simulink model "test_flock_gazebo"  (R2023b)
settings: Solver=FixedStepAuto  StartTime=0.0  StopTime=inf  RelTol=1e-3
values from neighbouring files (symbols this model uses):
  a = 1    [main_flock3.m]    (also in main_flock4.m; params_flocking_ros.m)
  b = 1    [main_flock3.m]    (also in main_flock4.m; params_flocking_ros.m)
  c = 1    [main_flock3.m]    (also in main_flock4.m; params_flocking_ros.m)
  c_gammap = 1.2    [main_flock3.m]    (also in main_flock4.m)
  c_gammav = 3.5    [main_flock3.m]    (also in main_flock4.m)
  d = 0.6    [main_flock3.m]    (also in main_flock4.m; params_flocking_ros.m)
  d_prime = 1    [main_flock3.m]    (also in main_flock4.m; params_flocking_ros.m)
  epsilon = 0.1    [main_flock3.m]    (also in main_flock4.m; params_flocking_ros.m)
  h = 0.2    [main_flock3.m]    (also in main_flock4.m; params_flocking_ros.m)
  R = 0.15    [main_flock3.m]    (also in main_flock4.m; params_flocking_ros.m)
  vxobs = 0    [main_flock3.m]    (also in main_flock4.m)
  vyobs = 0    [main_flock3.m]    (also in main_flock4.m)
  vzobs = 0    [main_flock3.m]    (also in main_flock4.m)
  xmax = 2    [main_flock3.m]    (also in main_flock4.m)
  xmin = -2    [main_flock3.m]    (also in main_flock4.m)
  xobs = 0.75    [main_flock3.m]    (also in main_flock4.m)
  yobs = -0.25    [main_flock3.m]    (also in main_flock4.m)
  zobs = 1.7    [main_flock3.m]    (also in main_flock4.m)
undefined symbols (not defined in the file or in its folder): angular, DiscIntNeverNeededParam, linear
libraries: ros2lib x14, robotcorelib x4
(part 1 of 2)
settings Model: Creator=johvany  LastModifiedBy=jonatan_alvarez
settings OptimizationCC: EnhancedBackFolding=on  PassReuseOutputArgsThreshold=0  ZeroExternalMemoryAtStartup=off  ZeroInternalMemoryAtStartup=off  MaxStackSize=64  OptimizeBlockOrder=speed  DifferentSizesBufferReuse=on  OptimizationCustomize=off
settings DebuggingCC: ParameterTunabilityLossMsg=error
settings HardwareCC: ProdBitPerLong=64  ProdHWDeviceType=Intel->x86-64 (Linux 64)  UseEmbeddedCoderFeatures=off
settings SFSimCC: MATLABDynamicMemAlloc=off
settings RTWCC: Description=Embedded Coder  SystemTargetFile=ert.tlc  HardwareBoard=Robot Operating System 2 (ROS 2)  TLCOptions="-aInlineSetEventsForThisBaseRateFcn=TLC_FALSE -aSuppressMultiTaskScheduler=TLC_FALSE  -aRateBasedStepFcn=0"  TemplateMakefile=ert_default_tmf  Toolchain=Colcon Tools  TargetLang=C++
settings CodeAppCC: ForceParamTrailComments=on  OperatorAnnotations=on
settings ERTTargetCC: ERTCustomFileBanners=off  CodeInterfacePackaging=C++ class  SupportContinuousTime=on  SupportNonInlinedSFcns=on  RemoveResetFunc=off  ModelStepFunctionPrototypeControlCompliant=off  RootIOFormat=Structure reference

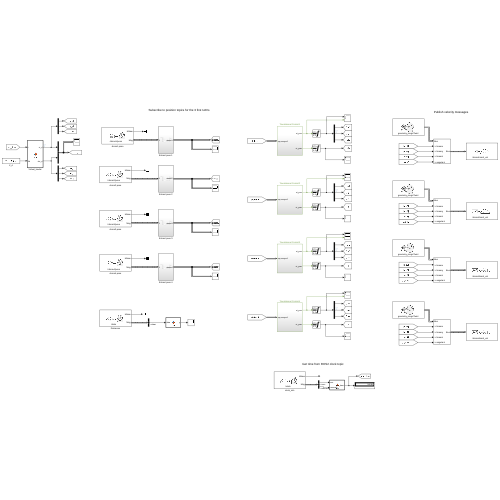
[thumbnail: Simulink's stored preview of the top-level diagram]
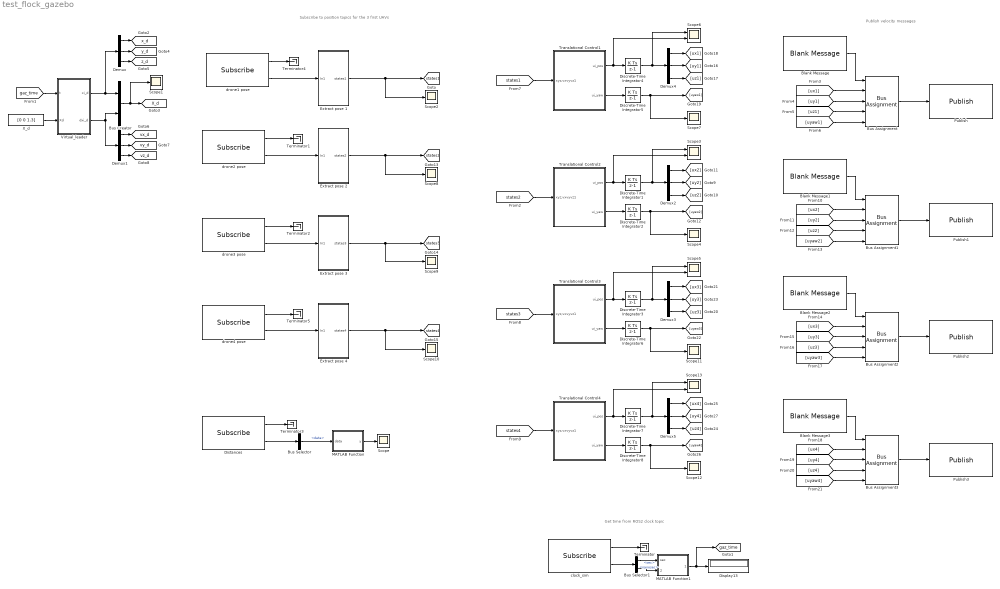
== system test_flock_gazebo ==
  note: Publish velocity messages
  note: Subscribe to position topics for the 3 first UAVs
  note: Get time from ROS2 clock topic
  Blank Message{,1..3} (4 alike) : ros2lib/Blank Message  messageClass=Message  entityType=geometry_msgs/Twist  messageType=geometry_msgs/Twist  SampleTime=inf
  Bus Assignment{,1..3} (4 alike) : BusAssignment  AssignedSignals=linear.x,linear.y,linear.z,angular.z
  Bus Creator : BusCreator  Inputs=2
  Bus Selector : BusSelector  OutputSignals=data
  Bus Selector1 : BusSelector  OutputSignals=clock.sec,clock.nanosec
  Demux{,1..5} (6 alike) : Demux  Outputs=3
  Discrete-Time Integrator{1..8} (8 alike) : DiscreteIntegrator  SampleTime=-1  LimitOutput=on  UpperSaturationLimit=5  LowerSaturationLimit=-5  ICPrevOutput=DiscIntNeverNeededParam  ICPrevScaledInput=DiscIntNeverNeededParam
  Display13 : Display
      settings: Decimation=4
  Distances : ros2lib/Subscribe  topicSource=Select from ROS network  topic=/dists  messageType=std_msgs/Float32MultiArray  sampleTime=-1  QOSHistory=Keep last  QOSDepth=1  QOSReliability=Reliable  QOSDurability=Volatile
  Extract pose 1 : Subsystem
  Extract pose 2 : Subsystem
  Extract pose 3 : Subsystem
  Extract pose 4 : Subsystem
  MATLAB Function : MATLAB Function  TreatAsAtomicUnit=on
  MATLAB Function1 : MATLAB Function  TreatAsAtomicUnit=on
  Publish : ros2lib/Publish  topicSource=Select from ROS network  topic=/drone1/cmd_vel  messageType=geometry_msgs/Twist  QOSHistory=Keep last  QOSDepth=1  QOSReliability=Reliable  QOSDurability=Volatile
  Publish1 : ros2lib/Publish  topicSource=Select from ROS network  topic=/drone2/cmd_vel  messageType=geometry_msgs/Twist  QOSHistory=Keep last  QOSDepth=1  QOSReliability=Reliable  QOSDurability=Volatile
  Publish2 : ros2lib/Publish  topicSource=Select from ROS network  topic=/drone3/cmd_vel  messageType=geometry_msgs/Twist  QOSHistory=Keep last  QOSDepth=1  QOSReliability=Reliable  QOSDurability=Volatile
  Publish3 : ros2lib/Publish  topicSource=Select from ROS network  topic=/drone4/cmd_vel  messageType=geometry_msgs/Twist  QOSHistory=Keep last  QOSDepth=1  QOSReliability=Reliable  QOSDurability=Volatile
  Scope{,1..2,4,7..12} (10 alike) : Scope
  Scope{3,5..6,13} (4 alike) : Scope  NumInputPorts=2
  Terminator{,1..5} (6 alike) : Terminator
  Translational Control1 : Subsystem
  Translational Control2 : Subsystem
  Translational Control3 : Subsystem
  Translational Control4 : Subsystem
  Virtual_leader : MATLAB Function  TreatAsAtomicUnit=on
  X_d : Constant  Value=[0 0 1.3]
  clock_sim : ros2lib/Subscribe  topicSource=Select from ROS network  topic=/clock  messageType=rosgraph_msgs/Clock  sampleTime=-1  QOSHistory=Keep last  QOSDepth=1  QOSReliability=Reliable  QOSDurability=Volatile
  drone1 pose : ros2lib/Subscribe  topicSource=Select from ROS network  topic=/drone1/pose  messageType=geometry_msgs/PoseStamped  sampleTime=-1  QOSHistory=Keep last  QOSDepth=1  QOSReliability=Reliable  QOSDurability=Volatile
  drone2 pose : ros2lib/Subscribe  topicSource=Select from ROS network  topic=/drone2/pose  messageType=geometry_msgs/PoseStamped  sampleTime=-1  QOSHistory=Keep last  QOSDepth=1  QOSReliability=Reliable  QOSDurability=Volatile
  drone3 pose : ros2lib/Subscribe  topicSource=Select from ROS network  topic=/drone3/pose  messageType=geometry_msgs/PoseStamped  sampleTime=-1  QOSHistory=Keep last  QOSDepth=1  QOSReliability=Reliable  QOSDurability=Volatile
  drone4 pose : ros2lib/Subscribe  topicSource=Select from ROS network  topic=/drone4/pose  messageType=geometry_msgs/PoseStamped  sampleTime=-1  QOSHistory=Keep last  QOSDepth=1  QOSReliability=Reliable  QOSDurability=Volatile
  tag scope: X_d=global, gaz_time=global, states1=global, states2=global, states3=global, states4=global, vx_d=global, vy_d=global, vz_d=global, x_d=global, y_d=global, z_d=global
  wires:
  clock_sim/1 -> Terminator/1
  drone2 pose/2 -> Extract pose 2/1(In1)
  drone2 pose/1 -> Terminator1/1
  drone3 pose/2 -> Extract pose 3/1(In1)
  drone3 pose/1 -> Terminator2/1
  Blank Message/1 -> Bus Assignment/1
  Bus Assignment/1 -> Publish/1
  Blank Message1/1 -> Bus Assignment1/1
  Bus Assignment1/1 -> Publish1/1
  Blank Message2/1 -> Bus Assignment2/1
  Bus Assignment2/1 -> Publish2/1
  Blank Message3/1 -> Bus Assignment3/1
  Bus Assignment3/1 -> Publish3/1
  Distances/1 -> Terminator3/1
  Distances/2 -> Bus Selector/1
  Bus Selector/1 -> MATLAB Function/1(data)  "<data>"
  MATLAB Function/1(y) -> Scope/1
  clock_sim/2 -> Bus Selector1/1
  Bus Selector1/1 -> MATLAB Function1/1(sec)  "<sec>"
  Bus Selector1/2 -> MATLAB Function1/2(nanosec)  "<nanosec>"
  Demux1/1 -> [vx_d]
  Demux1/3 -> [vz_d]
  Demux/1 -> [x_d]
  Demux/2 -> [y_d]
  Virtual_leader/2(dxi_d) -> Bus Creator/2, Demux1/1
  Bus Creator/1 -> Scope1/1, [X_d]
  Demux1/2 -> [vy_d]
  [gaz_time] -> Virtual_leader/1(t)
  Demux/3 -> [z_d]
  Virtual_leader/1(xi_d) -> Demux/1, Bus Creator/1
  drone1 pose/1 -> Terminator4/1
  drone1 pose/2 -> Extract pose 1/1(In1)
  MATLAB Function1/1(gaz_time) -> [gaz_time], Display13/1
  Extract pose 1/1(states1) -> [states1], Scope2/1
  [ux1] -> Bus Assignment/2
  [uy1] -> Bus Assignment/3
  [uz1] -> Bus Assignment/4
  [uyaw1] -> Bus Assignment/5
  X_d/1 -> Virtual_leader/2(Xd)
  [states1] -> Translational Control1/1(xyz,vxvyvz1)
  Translational Control1/1(ui_pos) -> Scope6/2, Discrete-Time Integrator4/1
  Translational Control1/2(ui_yaw) -> Discrete-Time Integrator5/1
  Discrete-Time Integrator5/1 -> [uyaw1], Scope7/1
  Extract pose 2/1(states2) -> Scope8/1, [states2]
  Extract pose 3/1(states3) -> [states3], Scope9/1
  Extract pose 4/1(states4) -> Scope10/1, [states4]
  drone4 pose/1 -> Terminator5/1
  drone4 pose/2 -> Extract pose 4/1(In1)
  Demux4/1 -> [ux1]
  Demux4/3 -> [uz1]
  Demux4/2 -> [uy1]
  Discrete-Time Integrator4/1 -> Scope6/1, Demux4/1
  Discrete-Time Integrator1/1 -> Demux2/1, Scope3/1
  Demux2/2 -> [uy2]
  Demux2/3 -> [uz2]
  Demux2/1 -> [ux2]
  Discrete-Time Integrator2/1 -> Scope4/1, [uyaw2]
  Translational Control2/2(ui_yaw) -> Discrete-Time Integrator2/1
  Translational Control2/1(ui_pos) -> Discrete-Time Integrator1/1, Scope3/2
  [states2] -> Translational Control2/1(xyz,vxvyvz1)
  [states3] -> Translational Control3/1(xyz,vxvyvz1)
  Translational Control3/1(ui_pos) -> Scope5/2, Discrete-Time Integrator3/1
  Translational Control3/2(ui_yaw) -> Discrete-Time Integrator6/1
  Discrete-Time Integrator6/1 -> [uyaw3], Scope11/1
  Demux3/1 -> [ux3]
  Demux3/3 -> [uz3]
  Demux3/2 -> [uy3]
  Discrete-Time Integrator3/1 -> Scope5/1, Demux3/1
  Discrete-Time Integrator7/1 -> Demux5/1, Scope13/1
  Demux5/2 -> [uy4]
  Demux5/3 -> [uz4]
  Demux5/1 -> [ux4]
  Discrete-Time Integrator8/1 -> Scope12/1, [uyaw4]
  Translational Control4/2(ui_yaw) -> Discrete-Time Integrator8/1
  Translational Control4/1(ui_pos) -> Discrete-Time Integrator7/1, Scope13/2
  [states4] -> Translational Control4/1(xyz,vxvyvz1)
  [ux2] -> Bus Assignment1/2
  [uy2] -> Bus Assignment1/3
  [uz2] -> Bus Assignment1/4
  [uyaw2] -> Bus Assignment1/5
  [uyaw3] -> Bus Assignment2/5
  [uz3] -> Bus Assignment2/4
  [uy3] -> Bus Assignment2/3
  [ux3] -> Bus Assignment2/2
  [ux4] -> Bus Assignment3/2
  [uy4] -> Bus Assignment3/3
  [uz4] -> Bus Assignment3/4
  [uyaw4] -> Bus Assignment3/5

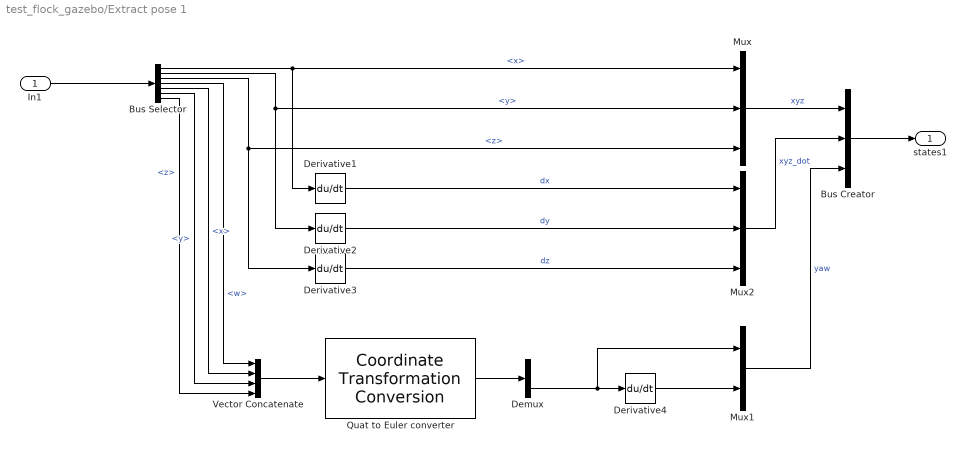
== system test_flock_gazebo/Extract pose 1 ==
  In1 : Inport
  Bus Creator : BusCreator  Inputs=3
  Bus Selector : BusSelector  OutputSignals=pose.position.x,pose.position.y,pose.position.z,pose.orientation.w,pose.orientation.x,pose.orientation.y,pose.orientation.z
  Demux : Demux  Outputs=3
  Derivative{1..4} (4 alike) : Derivative
  Mux : Mux  Inputs=3
  Mux1 : Mux  Inputs=2
  Mux2 : Mux  Inputs=3
  Quat to Euler converter : robotcorelib/Coordinate Transformation Conversion  InputRepresentation=Quaternion  InputEulerSequence=ZYX  ShowTrVecInputPort=on  OutputRepresentation=Euler Angles  OutputEulerSequence=XYZ  ShowTrVecOutputPort=on  SimulateUsing=Interpreted execution
      settings: LibrarySourceBlock=roslib/Utilities/Coordinate Transformation Conversion
  Vector Concatenate : Concatenate  NumInputs=4
  states1 : Outport
  wires:
  Bus Selector/5 -> Vector Concatenate/2  "<x>"
  Quat to Euler converter/1 -> Demux/1
  Demux/3 -> Mux1/1, Derivative4/1
  Bus Selector/6 -> Vector Concatenate/3  "<y>"
  Bus Selector/1 -> Derivative1/1, Mux/1  "<x>"
  Bus Selector/7 -> Vector Concatenate/4  "<z>"
  Vector Concatenate/1 -> Quat to Euler converter/1
  In1/1 -> Bus Selector/1
  Bus Selector/4 -> Vector Concatenate/1  "<w>"
  Bus Selector/2 -> Derivative2/1, Mux/2  "<y>"
  Bus Selector/3 -> Derivative3/1, Mux/3  "<z>"
  Derivative4/1 -> Mux1/2
  Bus Creator/1 -> states1/1
  Derivative1/1 -> Mux2/1  "dx"
  Derivative2/1 -> Mux2/2  "dy"
  Derivative3/1 -> Mux2/3  "dz"
  Mux/1 -> Bus Creator/1  "xyz"
  Mux2/1 -> Bus Creator/2  "xyz_dot"
  Mux1/1 -> Bus Creator/3  "yaw"

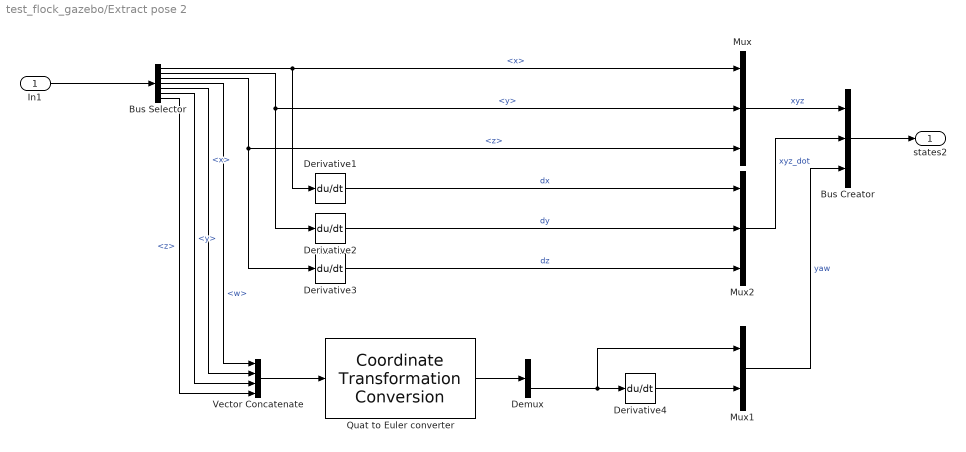
== system test_flock_gazebo/Extract pose 2 ==
  In1 : Inport
  Bus Creator : BusCreator  Inputs=3
  Bus Selector : BusSelector  OutputSignals=pose.position.x,pose.position.y,pose.position.z,pose.orientation.w,pose.orientation.x,pose.orientation.y,pose.orientation.z
  Demux : Demux  Outputs=3
  Derivative{1..4} (4 alike) : Derivative
  Mux : Mux  Inputs=3
  Mux1 : Mux  Inputs=2
  Mux2 : Mux  Inputs=3
  Quat to Euler converter : robotcorelib/Coordinate Transformation Conversion  InputRepresentation=Quaternion  InputEulerSequence=ZYX  ShowTrVecInputPort=on  OutputRepresentation=Euler Angles  OutputEulerSequence=XYZ  ShowTrVecOutputPort=on  SimulateUsing=Interpreted execution
      settings: LibrarySourceBlock=roslib/Utilities/Coordinate Transformation Conversion
  Vector Concatenate : Concatenate  NumInputs=4
  states2 : Outport
  wires:
  Mux1/1 -> Bus Creator/3  "yaw"
  Mux2/1 -> Bus Creator/2  "xyz_dot"
  Mux/1 -> Bus Creator/1  "xyz"
  Derivative3/1 -> Mux2/3  "dz"
  Derivative2/1 -> Mux2/2  "dy"
  Derivative1/1 -> Mux2/1  "dx"
  Bus Creator/1 -> states2/1
  Derivative4/1 -> Mux1/2
  Bus Selector/3 -> Mux/3, Derivative3/1  "<z>"
  Bus Selector/2 -> Mux/2, Derivative2/1  "<y>"
  Bus Selector/4 -> Vector Concatenate/1  "<w>"
  In1/1 -> Bus Selector/1
  Vector Concatenate/1 -> Quat to Euler converter/1
  Bus Selector/7 -> Vector Concatenate/4  "<z>"
  Bus Selector/1 -> Mux/1, Derivative1/1  "<x>"
  Bus Selector/6 -> Vector Concatenate/3  "<y>"
  Demux/3 -> Derivative4/1, Mux1/1
  Quat to Euler converter/1 -> Demux/1
  Bus Selector/5 -> Vector Concatenate/2  "<x>"

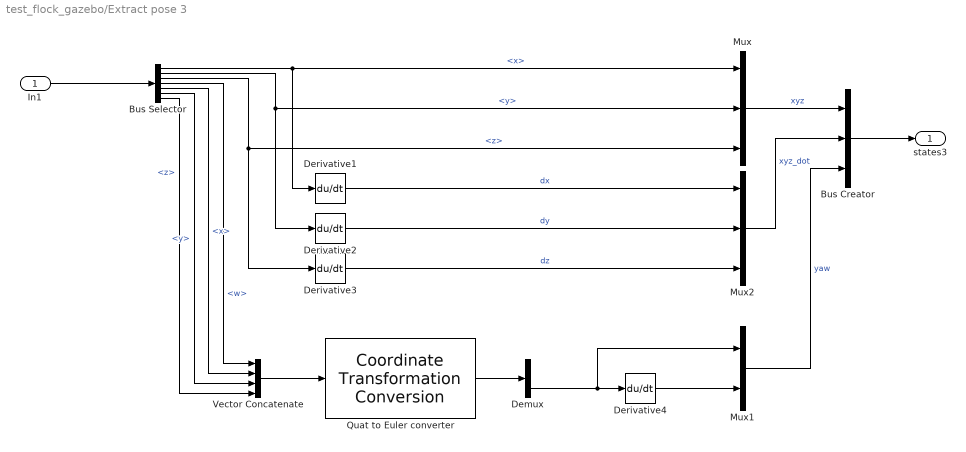
== system test_flock_gazebo/Extract pose 3 ==
  In1 : Inport
  Bus Creator : BusCreator  Inputs=3
  Bus Selector : BusSelector  OutputSignals=pose.position.x,pose.position.y,pose.position.z,pose.orientation.w,pose.orientation.x,pose.orientation.y,pose.orientation.z
  Demux : Demux  Outputs=3
  Derivative{1..4} (4 alike) : Derivative
  Mux : Mux  Inputs=3
  Mux1 : Mux  Inputs=2
  Mux2 : Mux  Inputs=3
  Quat to Euler converter : robotcorelib/Coordinate Transformation Conversion  InputRepresentation=Quaternion  InputEulerSequence=ZYX  ShowTrVecInputPort=on  OutputRepresentation=Euler Angles  OutputEulerSequence=XYZ  ShowTrVecOutputPort=on  SimulateUsing=Interpreted execution
      settings: LibrarySourceBlock=roslib/Utilities/Coordinate Transformation Conversion
  Vector Concatenate : Concatenate  NumInputs=4
  states3 : Outport
  wires:
  Bus Selector/5 -> Vector Concatenate/2  "<x>"
  Quat to Euler converter/1 -> Demux/1
  Demux/3 -> Mux1/1, Derivative4/1
  Bus Selector/6 -> Vector Concatenate/3  "<y>"
  Bus Selector/1 -> Derivative1/1, Mux/1  "<x>"
  Bus Selector/7 -> Vector Concatenate/4  "<z>"
  Vector Concatenate/1 -> Quat to Euler converter/1
  In1/1 -> Bus Selector/1
  Bus Selector/4 -> Vector Concatenate/1  "<w>"
  Bus Selector/2 -> Derivative2/1, Mux/2  "<y>"
  Bus Selector/3 -> Derivative3/1, Mux/3  "<z>"
  Derivative4/1 -> Mux1/2
  Bus Creator/1 -> states3/1
  Derivative1/1 -> Mux2/1  "dx"
  Derivative2/1 -> Mux2/2  "dy"
  Derivative3/1 -> Mux2/3  "dz"
  Mux/1 -> Bus Creator/1  "xyz"
  Mux2/1 -> Bus Creator/2  "xyz_dot"
  Mux1/1 -> Bus Creator/3  "yaw"

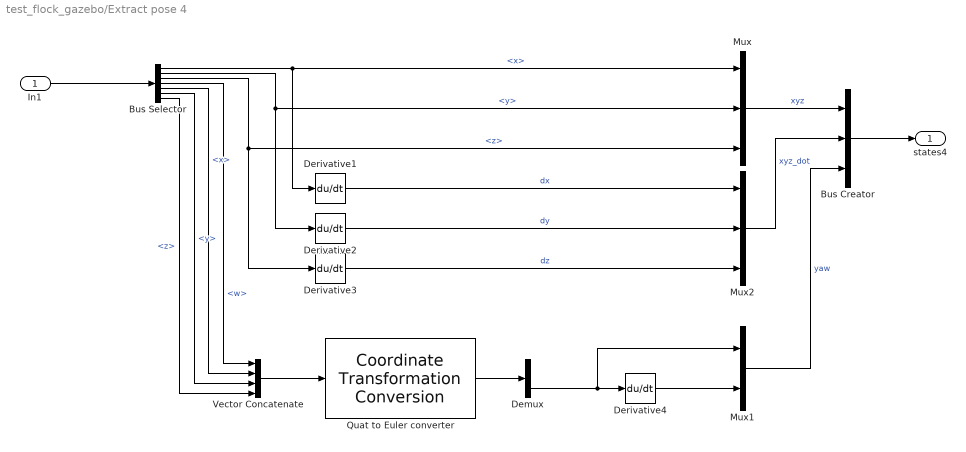
== system test_flock_gazebo/Extract pose 4 ==
  In1 : Inport
  Bus Creator : BusCreator  Inputs=3
  Bus Selector : BusSelector  OutputSignals=pose.position.x,pose.position.y,pose.position.z,pose.orientation.w,pose.orientation.x,pose.orientation.y,pose.orientation.z
  Demux : Demux  Outputs=3
  Derivative{1..4} (4 alike) : Derivative
  Mux : Mux  Inputs=3
  Mux1 : Mux  Inputs=2
  Mux2 : Mux  Inputs=3
  Quat to Euler converter : robotcorelib/Coordinate Transformation Conversion  InputRepresentation=Quaternion  InputEulerSequence=ZYX  ShowTrVecInputPort=on  OutputRepresentation=Euler Angles  OutputEulerSequence=XYZ  ShowTrVecOutputPort=on  SimulateUsing=Interpreted execution
      settings: LibrarySourceBlock=roslib/Utilities/Coordinate Transformation Conversion
  Vector Concatenate : Concatenate  NumInputs=4
  states4 : Outport
  wires:
  Mux1/1 -> Bus Creator/3  "yaw"
  Mux2/1 -> Bus Creator/2  "xyz_dot"
  Mux/1 -> Bus Creator/1  "xyz"
  Derivative3/1 -> Mux2/3  "dz"
  Derivative2/1 -> Mux2/2  "dy"
  Derivative1/1 -> Mux2/1  "dx"
  Bus Creator/1 -> states4/1
  Derivative4/1 -> Mux1/2
  Bus Selector/3 -> Mux/3, Derivative3/1  "<z>"
  Bus Selector/2 -> Mux/2, Derivative2/1  "<y>"
  Bus Selector/4 -> Vector Concatenate/1  "<w>"
  In1/1 -> Bus Selector/1
  Vector Concatenate/1 -> Quat to Euler converter/1
  Bus Selector/7 -> Vector Concatenate/4  "<z>"
  Bus Selector/1 -> Mux/1, Derivative1/1  "<x>"
  Bus Selector/6 -> Vector Concatenate/3  "<y>"
  Demux/3 -> Derivative4/1, Mux1/1
  Quat to Euler converter/1 -> Demux/1
  Bus Selector/5 -> Vector Concatenate/2  "<x>"

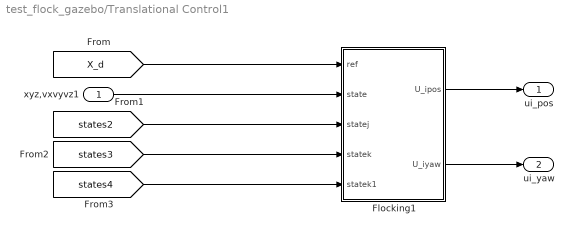
== system test_flock_gazebo/Translational Control1 ==
  xyz,vxvyvz1 : Inport
  Flocking1 : Subsystem
  ui_pos : Outport  VectorParamsAs1DForOutWhenUnconnected=off
  ui_yaw : Outport  Port=2  VectorParamsAs1DForOutWhenUnconnected=off
  wires:
  [X_d] -> Flocking1/1(ref)
  xyz,vxvyvz1/1 -> Flocking1/2(state)
  [states2] -> Flocking1/3(statej)
  [states3] -> Flocking1/4(statek)
  [states4] -> Flocking1/5(statek1)
  Flocking1/1(U_ipos) -> ui_pos/1
  Flocking1/2(U_iyaw) -> ui_yaw/1

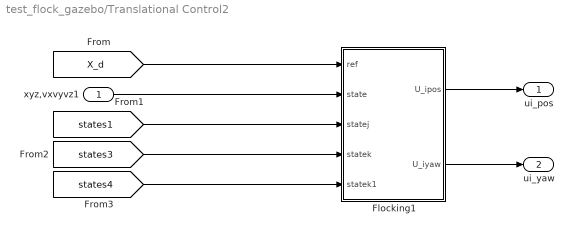
== system test_flock_gazebo/Translational Control2 ==
  xyz,vxvyvz1 : Inport
  Flocking1 : Subsystem
  ui_pos : Outport  VectorParamsAs1DForOutWhenUnconnected=off
  ui_yaw : Outport  Port=2  VectorParamsAs1DForOutWhenUnconnected=off
  wires:
  Flocking1/2(U_iyaw) -> ui_yaw/1
  Flocking1/1(U_ipos) -> ui_pos/1
  xyz,vxvyvz1/1 -> Flocking1/2(state)
  [X_d] -> Flocking1/1(ref)
  [states1] -> Flocking1/3(statej)
  [states3] -> Flocking1/4(statek)
  [states4] -> Flocking1/5(statek1)

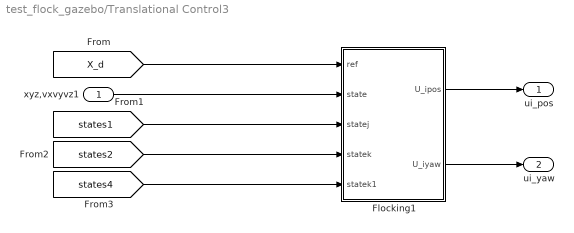
== system test_flock_gazebo/Translational Control3 ==
  xyz,vxvyvz1 : Inport
  Flocking1 : Subsystem
  ui_pos : Outport  VectorParamsAs1DForOutWhenUnconnected=off
  ui_yaw : Outport  Port=2  VectorParamsAs1DForOutWhenUnconnected=off
  wires:
  [states4] -> Flocking1/5(statek1)
  [states2] -> Flocking1/4(statek)
  [states1] -> Flocking1/3(statej)
  [X_d] -> Flocking1/1(ref)
  xyz,vxvyvz1/1 -> Flocking1/2(state)
  Flocking1/1(U_ipos) -> ui_pos/1
  Flocking1/2(U_iyaw) -> ui_yaw/1

== system test_flock_gazebo/Translational Control4 ==
  xyz,vxvyvz1 : Inport
  Flocking1 : Subsystem
  ui_pos : Outport  VectorParamsAs1DForOutWhenUnconnected=off
  ui_yaw : Outport  Port=2  VectorParamsAs1DForOutWhenUnconnected=off
  wires:
  Flocking1/2(U_iyaw) -> ui_yaw/1
  Flocking1/1(U_ipos) -> ui_pos/1
  xyz,vxvyvz1/1 -> Flocking1/2(state)
  [X_d] -> Flocking1/1(ref)
  [states1] -> Flocking1/3(statej)
  [states2] -> Flocking1/4(statek)
  [states3] -> Flocking1/5(statek1)

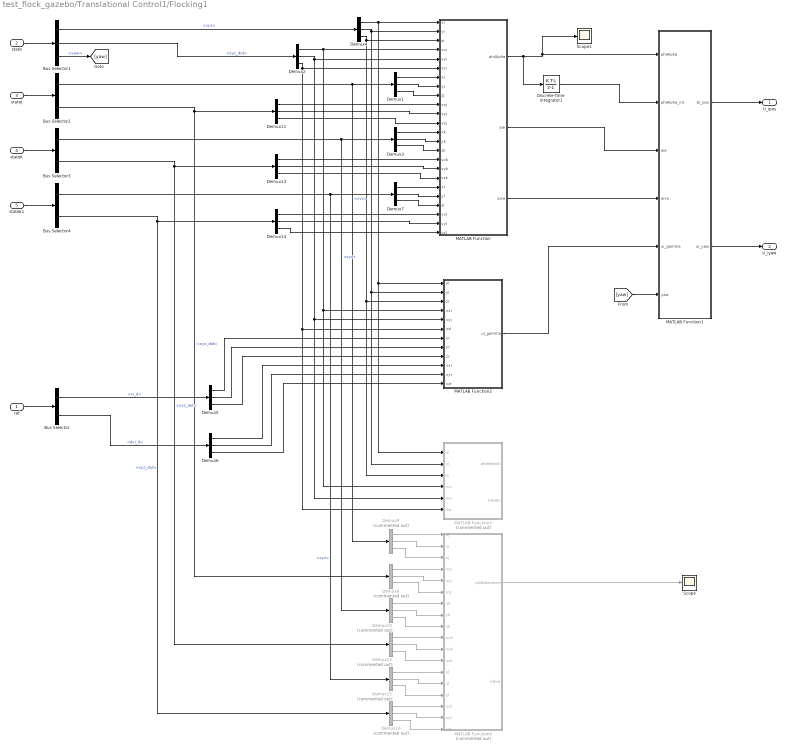
== system test_flock_gazebo/Translational Control1/Flocking1 ==
  ref : Inport
  state : Inport  Port=2
  statej : Inport  Port=3
  statek : Inport  Port=4
  statek1 : Inport  Port=5
  Bus Selector : BusSelector  OutputSignals=xi_d,dxi_d
  Bus Selector1 : BusSelector  OutputSignals=xyz,xyz_dot,yaw
  Bus Selector2 : BusSelector  OutputSignals=xyz,xyz_dot
  Bus Selector3 : BusSelector  OutputSignals=xyz,xyz_dot
  Bus Selector4 : BusSelector  OutputSignals=xyz,xyz_dot
  Demux{1..7,11,13..14} (10 alike) : Demux  Outputs=3
  Demux{8..10,12,15..16} (6 alike) : Demux  Commented=on  Outputs=3
  Discrete-Time Integrator1 : DiscreteIntegrator  SampleTime=-1  LimitOutput=on  UpperSaturationLimit=5  LowerSaturationLimit=-5  ICPrevOutput=DiscIntNeverNeededParam  ICPrevScaledInput=DiscIntNeverNeededParam
  MATLAB Function : MATLAB Function  TreatAsAtomicUnit=on
  MATLAB Function1 : MATLAB Function  TreatAsAtomicUnit=on
  MATLAB Function2 : MATLAB Function  TreatAsAtomicUnit=on
  MATLAB Function3 : MATLAB Function  Commented=on  TreatAsAtomicUnit=on
  MATLAB Function4 : MATLAB Function  Commented=on  TreatAsAtomicUnit=on
  Scope : Scope
  Scope1 : Scope
  U_ipos : Outport  VectorParamsAs1DForOutWhenUnconnected=off
  U_iyaw : Outport  Port=2  VectorParamsAs1DForOutWhenUnconnected=off
  wires:
  ref/1 -> Bus Selector/1
  state/1 -> Bus Selector1/1
  Bus Selector/2 -> Demux6/1  "<dxi_d>"
  Bus Selector/1 -> Demux5/1  "<xi_d>"
  Demux6/1 -> MATLAB Function2/10(vxr)
  Demux6/2 -> MATLAB Function2/11(vyr)
  statej/1 -> Bus Selector2/1
  Bus Selector2/1 -> Demux9/1, Demux1/1  "<xyz>"
  Demux4/1 -> MATLAB Function3/1(xi), MATLAB Function2/1(xi), MATLAB Function/1(xi)
  Demux4/2 -> MATLAB Function3/2(yi), MATLAB Function2/2(yi), MATLAB Function/2(yi)
  Demux1/1 -> MATLAB Function/7(xj)
  Demux1/2 -> MATLAB Function/8(yj)
  Bus Selector2/2 -> Demux8/1, Demux11/1  "<xyz_dot>"
  Discrete-Time Integrator1/1 -> MATLAB Function1/2(phiAlpha_int)
  MATLAB Function2/1(ui_gamma) -> MATLAB Function1/5(ui_gamma)
  statek/1 -> Bus Selector3/1
  Bus Selector3/2 -> Demux12/1, Demux13/1  "<xyz_dot>"
  Demux3/1 -> MATLAB Function/13(xk)
  Demux3/2 -> MATLAB Function/14(yk)
  Bus Selector3/1 -> Demux10/1, Demux3/1  "<xyz>"
  Demux9/1 -> MATLAB Function4/1(xj)
  Demux9/2 -> MATLAB Function4/2(yj)
  Demux10/1 -> MATLAB Function4/7(xk)
  Demux10/2 -> MATLAB Function4/8(yk)
  MATLAB Function/1(phiAlpha) -> Discrete-Time Integrator1/1, Scope1/1, MATLAB Function1/1(phiAlpha)
  Demux5/1 -> MATLAB Function2/7(xr)
  Demux5/2 -> MATLAB Function2/8(yr)
  Demux4/3 -> MATLAB Function3/3(zi), MATLAB Function2/3(zi), MATLAB Function/3(zi)
  Demux3/3 -> MATLAB Function/15(zk)
  Demux5/3 -> MATLAB Function2/9(zr)
  Demux6/3 -> MATLAB Function2/12(vzr)
  MATLAB Function1/1(Ui_pos) -> U_ipos/1
  Demux2/1 -> MATLAB Function2/4(vxi), MATLAB Function3/4(vxi), MATLAB Function/4(vxi)
  Demux2/2 -> MATLAB Function3/5(vyi), MATLAB Function2/5(vyi), MATLAB Function/5(vyi)
  Demux2/3 -> MATLAB Function3/6(vzi), MATLAB Function2/6(vzi), MATLAB Function/6(vzi)
  Demux1/3 -> MATLAB Function/9(zj)
  Demux11/1 -> MATLAB Function/10(vxj)
  Demux11/2 -> MATLAB Function/11(vyj)
  Demux11/3 -> MATLAB Function/12(vzj)
  Demux13/1 -> MATLAB Function/16(vxk)
  Demux13/2 -> MATLAB Function/17(vyk)
  Demux13/3 -> MATLAB Function/18(vzk)
  MATLAB Function/3(aive) -> MATLAB Function1/4(aive)
  Demux9/3 -> MATLAB Function4/3(zj)
  Demux10/3 -> MATLAB Function4/9(zk)
  MATLAB Function4/1(phiBetaniknei) -> Scope/1
  Demux8/1 -> MATLAB Function4/4(vxj)
  Demux8/2 -> MATLAB Function4/5(vyj)
  Demux8/3 -> MATLAB Function4/6(vzj)
  Demux12/1 -> MATLAB Function4/10(vxk)
  Demux12/2 -> MATLAB Function4/11(vyk)
  Demux12/3 -> MATLAB Function4/12(vzk)
  MATLAB Function/2(aie) -> MATLAB Function1/3(aie)
  statek1/1 -> Bus Selector4/1
  Demux7/1 -> MATLAB Function/19(xl)
  Demux7/2 -> MATLAB Function/20(yl)
  Demux7/3 -> MATLAB Function/21(zl)
  Bus Selector4/1 -> Demux15/1, Demux7/1  "<xyz>"
  Demux14/1 -> MATLAB Function/22(vxl)
  Demux14/2 -> MATLAB Function/23(vyl)
  Demux14/3 -> MATLAB Function/24(vzl)
  Bus Selector4/2 -> Demux16/1, Demux14/1  "<xyz_dot>"
  Demux15/1 -> MATLAB Function4/13(xl)
  Demux15/2 -> MATLAB Function4/14(yl)
  Demux15/3 -> MATLAB Function4/15(zl)
  Demux16/1 -> MATLAB Function4/16(vxl)
  Demux16/2 -> MATLAB Function4/17(vyl)
  Demux16/3 -> MATLAB Function4/18(vzl)
  Bus Selector1/1 -> Demux4/1  "<xyz>"
  Bus Selector1/2 -> Demux2/1  "<xyz_dot>"
  Bus Selector1/3 -> [yaw]  "<yaw>"
  [yaw] -> MATLAB Function1/6(yaw)
  MATLAB Function1/2(ui_yaw) -> U_iyaw/1

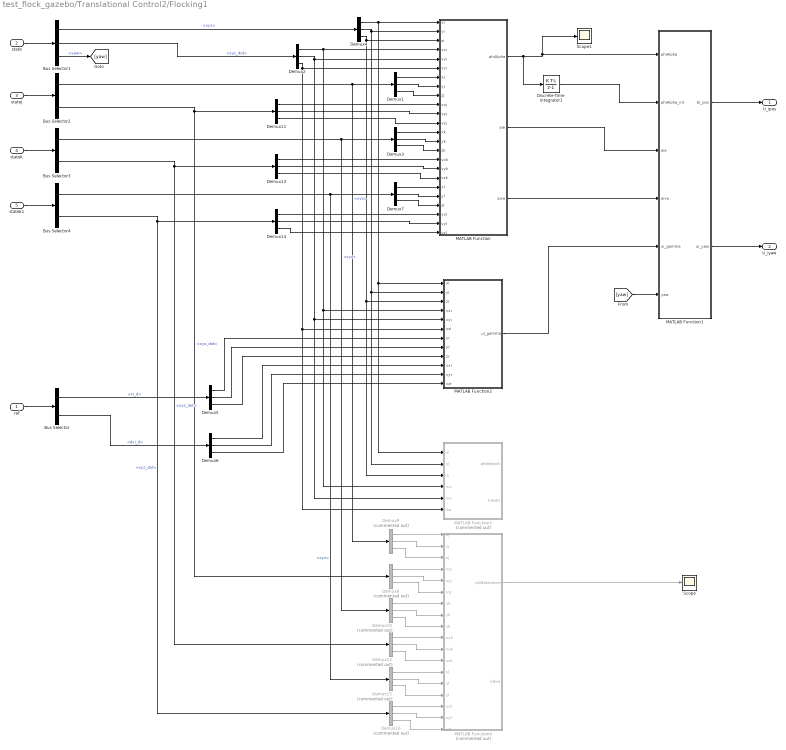
== system test_flock_gazebo/Translational Control2/Flocking1 ==
  ref : Inport
  state : Inport  Port=2
  statej : Inport  Port=3
  statek : Inport  Port=4
  statek1 : Inport  Port=5
  Bus Selector : BusSelector  OutputSignals=xi_d,dxi_d
  Bus Selector1 : BusSelector  OutputSignals=xyz,xyz_dot,yaw
  Bus Selector2 : BusSelector  OutputSignals=xyz,xyz_dot
  Bus Selector3 : BusSelector  OutputSignals=xyz,xyz_dot
  Bus Selector4 : BusSelector  OutputSignals=xyz,xyz_dot
  Demux{1..7,11,13..14} (10 alike) : Demux  Outputs=3
  Demux{8..10,12,15..16} (6 alike) : Demux  Commented=on  Outputs=3
  Discrete-Time Integrator1 : DiscreteIntegrator  SampleTime=-1  LimitOutput=on  UpperSaturationLimit=5  LowerSaturationLimit=-5  ICPrevOutput=DiscIntNeverNeededParam  ICPrevScaledInput=DiscIntNeverNeededParam
  MATLAB Function : MATLAB Function  TreatAsAtomicUnit=on
  MATLAB Function1 : MATLAB Function  TreatAsAtomicUnit=on
  MATLAB Function2 : MATLAB Function  TreatAsAtomicUnit=on
  MATLAB Function3 : MATLAB Function  Commented=on  TreatAsAtomicUnit=on
  MATLAB Function4 : MATLAB Function  Commented=on  TreatAsAtomicUnit=on
  Scope : Scope
  Scope1 : Scope
  U_ipos : Outport  VectorParamsAs1DForOutWhenUnconnected=off
  U_iyaw : Outport  Port=2  VectorParamsAs1DForOutWhenUnconnected=off
  wires:
  MATLAB Function1/2(ui_yaw) -> U_iyaw/1
  [yaw] -> MATLAB Function1/6(yaw)
  Bus Selector1/3 -> [yaw]  "<yaw>"
  Bus Selector1/2 -> Demux2/1  "<xyz_dot>"
  Bus Selector1/1 -> Demux4/1  "<xyz>"
  Demux16/3 -> MATLAB Function4/18(vzl)
  Demux16/2 -> MATLAB Function4/17(vyl)
  Demux16/1 -> MATLAB Function4/16(vxl)
  Demux15/3 -> MATLAB Function4/15(zl)
  Demux15/2 -> MATLAB Function4/14(yl)
  Demux15/1 -> MATLAB Function4/13(xl)
  Bus Selector4/2 -> Demux14/1, Demux16/1  "<xyz_dot>"
  Demux14/3 -> MATLAB Function/24(vzl)
  Demux14/2 -> MATLAB Function/23(vyl)
  Demux14/1 -> MATLAB Function/22(vxl)
  Bus Selector4/1 -> Demux7/1, Demux15/1  "<xyz>"
  Demux7/3 -> MATLAB Function/21(zl)
  Demux7/2 -> MATLAB Function/20(yl)
  Demux7/1 -> MATLAB Function/19(xl)
  statek1/1 -> Bus Selector4/1
  MATLAB Function/2(aie) -> MATLAB Function1/3(aie)
  Demux12/3 -> MATLAB Function4/12(vzk)
  Demux12/2 -> MATLAB Function4/11(vyk)
  Demux12/1 -> MATLAB Function4/10(vxk)
  Demux8/3 -> MATLAB Function4/6(vzj)
  Demux8/2 -> MATLAB Function4/5(vyj)
  Demux8/1 -> MATLAB Function4/4(vxj)
  MATLAB Function4/1(phiBetaniknei) -> Scope/1
  Demux10/3 -> MATLAB Function4/9(zk)
  Demux9/3 -> MATLAB Function4/3(zj)
  MATLAB Function/3(aive) -> MATLAB Function1/4(aive)
  Demux13/3 -> MATLAB Function/18(vzk)
  Demux13/2 -> MATLAB Function/17(vyk)
  Demux13/1 -> MATLAB Function/16(vxk)
  Demux11/3 -> MATLAB Function/12(vzj)
  Demux11/2 -> MATLAB Function/11(vyj)
  Demux11/1 -> MATLAB Function/10(vxj)
  Demux1/3 -> MATLAB Function/9(zj)
  Demux2/3 -> MATLAB Function/6(vzi), MATLAB Function2/6(vzi), MATLAB Function3/6(vzi)
  Demux2/2 -> MATLAB Function/5(vyi), MATLAB Function2/5(vyi), MATLAB Function3/5(vyi)
  Demux2/1 -> MATLAB Function/4(vxi), MATLAB Function3/4(vxi), MATLAB Function2/4(vxi)
  MATLAB Function1/1(Ui_pos) -> U_ipos/1
  Demux6/3 -> MATLAB Function2/12(vzr)
  Demux5/3 -> MATLAB Function2/9(zr)
  Demux3/3 -> MATLAB Function/15(zk)
  Demux4/3 -> MATLAB Function/3(zi), MATLAB Function2/3(zi), MATLAB Function3/3(zi)
  Demux5/2 -> MATLAB Function2/8(yr)
  Demux5/1 -> MATLAB Function2/7(xr)
  MATLAB Function/1(phiAlpha) -> MATLAB Function1/1(phiAlpha), Scope1/1, Discrete-Time Integrator1/1
  Demux10/2 -> MATLAB Function4/8(yk)
  Demux10/1 -> MATLAB Function4/7(xk)
  Demux9/2 -> MATLAB Function4/2(yj)
  Demux9/1 -> MATLAB Function4/1(xj)
  Bus Selector3/1 -> Demux3/1, Demux10/1  "<xyz>"
  Demux3/2 -> MATLAB Function/14(yk)
  Demux3/1 -> MATLAB Function/13(xk)
  Bus Selector3/2 -> Demux13/1, Demux12/1  "<xyz_dot>"
  statek/1 -> Bus Selector3/1
  MATLAB Function2/1(ui_gamma) -> MATLAB Function1/5(ui_gamma)
  Discrete-Time Integrator1/1 -> MATLAB Function1/2(phiAlpha_int)
  Bus Selector2/2 -> Demux11/1, Demux8/1  "<xyz_dot>"
  Demux1/2 -> MATLAB Function/8(yj)
  Demux1/1 -> MATLAB Function/7(xj)
  Demux4/2 -> MATLAB Function/2(yi), MATLAB Function2/2(yi), MATLAB Function3/2(yi)
  Demux4/1 -> MATLAB Function/1(xi), MATLAB Function2/1(xi), MATLAB Function3/1(xi)
  Bus Selector2/1 -> Demux1/1, Demux9/1  "<xyz>"
  statej/1 -> Bus Selector2/1
  Demux6/2 -> MATLAB Function2/11(vyr)
  Demux6/1 -> MATLAB Function2/10(vxr)
  Bus Selector/1 -> Demux5/1  "<xi_d>"
  Bus Selector/2 -> Demux6/1  "<dxi_d>"
  state/1 -> Bus Selector1/1
  ref/1 -> Bus Selector/1

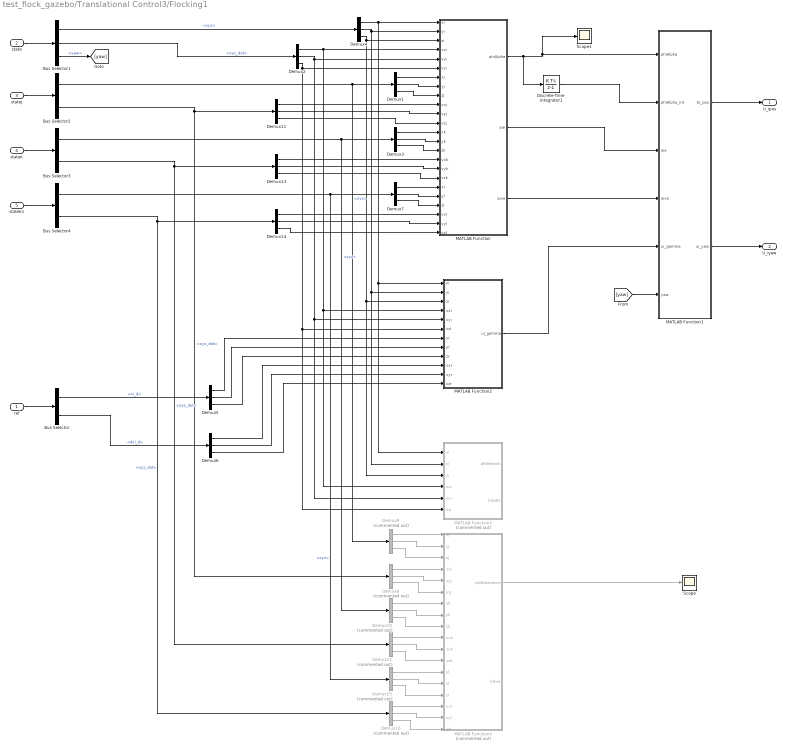
== system test_flock_gazebo/Translational Control3/Flocking1 ==
  ref : Inport
  state : Inport  Port=2
  statej : Inport  Port=3
  statek : Inport  Port=4
  statek1 : Inport  Port=5
  Bus Selector : BusSelector  OutputSignals=xi_d,dxi_d
  Bus Selector1 : BusSelector  OutputSignals=xyz,xyz_dot,yaw
  Bus Selector2 : BusSelector  OutputSignals=xyz,xyz_dot
  Bus Selector3 : BusSelector  OutputSignals=xyz,xyz_dot
  Bus Selector4 : BusSelector  OutputSignals=xyz,xyz_dot
  Demux{1..7,11,13..14} (10 alike) : Demux  Outputs=3
  Demux{8..10,12,15..16} (6 alike) : Demux  Commented=on  Outputs=3
  Discrete-Time Integrator1 : DiscreteIntegrator  SampleTime=-1  LimitOutput=on  UpperSaturationLimit=5  LowerSaturationLimit=-5  ICPrevOutput=DiscIntNeverNeededParam  ICPrevScaledInput=DiscIntNeverNeededParam
  MATLAB Function : MATLAB Function  TreatAsAtomicUnit=on
  MATLAB Function1 : MATLAB Function  TreatAsAtomicUnit=on
  MATLAB Function2 : MATLAB Function  TreatAsAtomicUnit=on
  MATLAB Function3 : MATLAB Function  Commented=on  TreatAsAtomicUnit=on
  MATLAB Function4 : MATLAB Function  Commented=on  TreatAsAtomicUnit=on
  Scope : Scope
  Scope1 : Scope
  U_ipos : Outport  VectorParamsAs1DForOutWhenUnconnected=off
  U_iyaw : Outport  Port=2  VectorParamsAs1DForOutWhenUnconnected=off
  wires:
  ref/1 -> Bus Selector/1
  state/1 -> Bus Selector1/1
  Bus Selector/2 -> Demux6/1  "<dxi_d>"
  Bus Selector/1 -> Demux5/1  "<xi_d>"
  Demux6/1 -> MATLAB Function2/10(vxr)
  Demux6/2 -> MATLAB Function2/11(vyr)
  statej/1 -> Bus Selector2/1
  Bus Selector2/1 -> Demux9/1, Demux1/1  "<xyz>"
  Demux4/1 -> MATLAB Function3/1(xi), MATLAB Function2/1(xi), MATLAB Function/1(xi)
  Demux4/2 -> MATLAB Function3/2(yi), MATLAB Function2/2(yi), MATLAB Function/2(yi)
  Demux1/1 -> MATLAB Function/7(xj)
  Demux1/2 -> MATLAB Function/8(yj)
  Bus Selector2/2 -> Demux8/1, Demux11/1  "<xyz_dot>"
  Discrete-Time Integrator1/1 -> MATLAB Function1/2(phiAlpha_int)
  MATLAB Function2/1(ui_gamma) -> MATLAB Function1/5(ui_gamma)
  statek/1 -> Bus Selector3/1
  Bus Selector3/2 -> Demux12/1, Demux13/1  "<xyz_dot>"
  Demux3/1 -> MATLAB Function/13(xk)
  Demux3/2 -> MATLAB Function/14(yk)
  Bus Selector3/1 -> Demux10/1, Demux3/1  "<xyz>"
  Demux9/1 -> MATLAB Function4/1(xj)
  Demux9/2 -> MATLAB Function4/2(yj)
  Demux10/1 -> MATLAB Function4/7(xk)
  Demux10/2 -> MATLAB Function4/8(yk)
  MATLAB Function/1(phiAlpha) -> Discrete-Time Integrator1/1, Scope1/1, MATLAB Function1/1(phiAlpha)
  Demux5/1 -> MATLAB Function2/7(xr)
  Demux5/2 -> MATLAB Function2/8(yr)
  Demux4/3 -> MATLAB Function3/3(zi), MATLAB Function2/3(zi), MATLAB Function/3(zi)
  Demux3/3 -> MATLAB Function/15(zk)
  Demux5/3 -> MATLAB Function2/9(zr)
  Demux6/3 -> MATLAB Function2/12(vzr)
  MATLAB Function1/1(Ui_pos) -> U_ipos/1
  Demux2/1 -> MATLAB Function2/4(vxi), MATLAB Function3/4(vxi), MATLAB Function/4(vxi)
  Demux2/2 -> MATLAB Function3/5(vyi), MATLAB Function2/5(vyi), MATLAB Function/5(vyi)
  Demux2/3 -> MATLAB Function3/6(vzi), MATLAB Function2/6(vzi), MATLAB Function/6(vzi)
  Demux1/3 -> MATLAB Function/9(zj)
  Demux11/1 -> MATLAB Function/10(vxj)
  Demux11/2 -> MATLAB Function/11(vyj)
  Demux11/3 -> MATLAB Function/12(vzj)
  Demux13/1 -> MATLAB Function/16(vxk)
  Demux13/2 -> MATLAB Function/17(vyk)
  Demux13/3 -> MATLAB Function/18(vzk)
  MATLAB Function/3(aive) -> MATLAB Function1/4(aive)
  Demux9/3 -> MATLAB Function4/3(zj)
  Demux10/3 -> MATLAB Function4/9(zk)
  MATLAB Function4/1(phiBetaniknei) -> Scope/1
  Demux8/1 -> MATLAB Function4/4(vxj)
  Demux8/2 -> MATLAB Function4/5(vyj)
  Demux8/3 -> MATLAB Function4/6(vzj)
  Demux12/1 -> MATLAB Function4/10(vxk)
  Demux12/2 -> MATLAB Function4/11(vyk)
  Demux12/3 -> MATLAB Function4/12(vzk)
  MATLAB Function/2(aie) -> MATLAB Function1/3(aie)
  statek1/1 -> Bus Selector4/1
  Demux7/1 -> MATLAB Function/19(xl)
  Demux7/2 -> MATLAB Function/20(yl)
  Demux7/3 -> MATLAB Function/21(zl)
  Bus Selector4/1 -> Demux15/1, Demux7/1  "<xyz>"
  Demux14/1 -> MATLAB Function/22(vxl)
  Demux14/2 -> MATLAB Function/23(vyl)
  Demux14/3 -> MATLAB Function/24(vzl)
  Bus Selector4/2 -> Demux16/1, Demux14/1  "<xyz_dot>"
  Demux15/1 -> MATLAB Function4/13(xl)
  Demux15/2 -> MATLAB Function4/14(yl)
  Demux15/3 -> MATLAB Function4/15(zl)
  Demux16/1 -> MATLAB Function4/16(vxl)
  Demux16/2 -> MATLAB Function4/17(vyl)
  Demux16/3 -> MATLAB Function4/18(vzl)
  Bus Selector1/1 -> Demux4/1  "<xyz>"
  Bus Selector1/2 -> Demux2/1  "<xyz_dot>"
  Bus Selector1/3 -> [yaw]  "<yaw>"
  [yaw] -> MATLAB Function1/6(yaw)
  MATLAB Function1/2(ui_yaw) -> U_iyaw/1

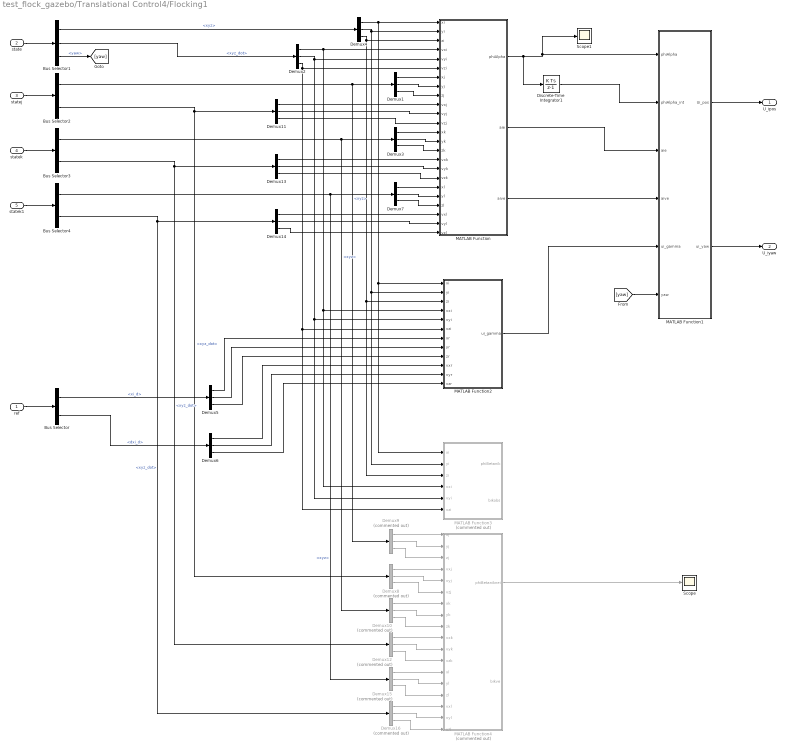
== system test_flock_gazebo/Translational Control4/Flocking1 ==
  ref : Inport
  state : Inport  Port=2
  statej : Inport  Port=3
  statek : Inport  Port=4
  statek1 : Inport  Port=5
  Bus Selector : BusSelector  OutputSignals=xi_d,dxi_d
  Bus Selector1 : BusSelector  OutputSignals=xyz,xyz_dot,yaw
  Bus Selector2 : BusSelector  OutputSignals=xyz,xyz_dot
  Bus Selector3 : BusSelector  OutputSignals=xyz,xyz_dot
  Bus Selector4 : BusSelector  OutputSignals=xyz,xyz_dot
  Demux{1..7,11,13..14} (10 alike) : Demux  Outputs=3
  Demux{8..10,12,15..16} (6 alike) : Demux  Commented=on  Outputs=3
  Discrete-Time Integrator1 : DiscreteIntegrator  SampleTime=-1  LimitOutput=on  UpperSaturationLimit=5  LowerSaturationLimit=-5  ICPrevOutput=DiscIntNeverNeededParam  ICPrevScaledInput=DiscIntNeverNeededParam
  MATLAB Function : MATLAB Function  TreatAsAtomicUnit=on
  MATLAB Function1 : MATLAB Function  TreatAsAtomicUnit=on
  MATLAB Function2 : MATLAB Function  TreatAsAtomicUnit=on
  MATLAB Function3 : MATLAB Function  Commented=on  TreatAsAtomicUnit=on
  MATLAB Function4 : MATLAB Function  Commented=on  TreatAsAtomicUnit=on
  Scope : Scope
  Scope1 : Scope
  U_ipos : Outport  VectorParamsAs1DForOutWhenUnconnected=off
  U_iyaw : Outport  Port=2  VectorParamsAs1DForOutWhenUnconnected=off
  wires:
  MATLAB Function1/2(ui_yaw) -> U_iyaw/1
  [yaw] -> MATLAB Function1/6(yaw)
  Bus Selector1/3 -> [yaw]  "<yaw>"
  Bus Selector1/2 -> Demux2/1  "<xyz_dot>"
  Bus Selector1/1 -> Demux4/1  "<xyz>"
  Demux16/3 -> MATLAB Function4/18(vzl)
  Demux16/2 -> MATLAB Function4/17(vyl)
  Demux16/1 -> MATLAB Function4/16(vxl)
  Demux15/3 -> MATLAB Function4/15(zl)
  Demux15/2 -> MATLAB Function4/14(yl)
  Demux15/1 -> MATLAB Function4/13(xl)
  Bus Selector4/2 -> Demux14/1, Demux16/1  "<xyz_dot>"
  Demux14/3 -> MATLAB Function/24(vzl)
  Demux14/2 -> MATLAB Function/23(vyl)
  Demux14/1 -> MATLAB Function/22(vxl)
  Bus Selector4/1 -> Demux7/1, Demux15/1  "<xyz>"
  Demux7/3 -> MATLAB Function/21(zl)
  Demux7/2 -> MATLAB Function/20(yl)
  Demux7/1 -> MATLAB Function/19(xl)
  statek1/1 -> Bus Selector4/1
  MATLAB Function/2(aie) -> MATLAB Function1/3(aie)
  Demux12/3 -> MATLAB Function4/12(vzk)
  Demux12/2 -> MATLAB Function4/11(vyk)
  Demux12/1 -> MATLAB Function4/10(vxk)
  Demux8/3 -> MATLAB Function4/6(vzj)
  Demux8/2 -> MATLAB Function4/5(vyj)
  Demux8/1 -> MATLAB Function4/4(vxj)
  MATLAB Function4/1(phiBetaniknei) -> Scope/1
  Demux10/3 -> MATLAB Function4/9(zk)
  Demux9/3 -> MATLAB Function4/3(zj)
  MATLAB Function/3(aive) -> MATLAB Function1/4(aive)
  Demux13/3 -> MATLAB Function/18(vzk)
  Demux13/2 -> MATLAB Function/17(vyk)
  Demux13/1 -> MATLAB Function/16(vxk)
  Demux11/3 -> MATLAB Function/12(vzj)
  Demux11/2 -> MATLAB Function/11(vyj)
  Demux11/1 -> MATLAB Function/10(vxj)
  Demux1/3 -> MATLAB Function/9(zj)
  Demux2/3 -> MATLAB Function/6(vzi), MATLAB Function2/6(vzi), MATLAB Function3/6(vzi)
  Demux2/2 -> MATLAB Function/5(vyi), MATLAB Function2/5(vyi), MATLAB Function3/5(vyi)
  Demux2/1 -> MATLAB Function/4(vxi), MATLAB Function3/4(vxi), MATLAB Function2/4(vxi)
  MATLAB Function1/1(Ui_pos) -> U_ipos/1
  Demux6/3 -> MATLAB Function2/12(vzr)
  Demux5/3 -> MATLAB Function2/9(zr)
  Demux3/3 -> MATLAB Function/15(zk)
  Demux4/3 -> MATLAB Function/3(zi), MATLAB Function2/3(zi), MATLAB Function3/3(zi)
  Demux5/2 -> MATLAB Function2/8(yr)
  Demux5/1 -> MATLAB Function2/7(xr)
  MATLAB Function/1(phiAlpha) -> MATLAB Function1/1(phiAlpha), Scope1/1, Discrete-Time Integrator1/1
  Demux10/2 -> MATLAB Function4/8(yk)
  Demux10/1 -> MATLAB Function4/7(xk)
  Demux9/2 -> MATLAB Function4/2(yj)
  Demux9/1 -> MATLAB Function4/1(xj)
  Bus Selector3/1 -> Demux3/1, Demux10/1  "<xyz>"
  Demux3/2 -> MATLAB Function/14(yk)
  Demux3/1 -> MATLAB Function/13(xk)
  Bus Selector3/2 -> Demux13/1, Demux12/1  "<xyz_dot>"
  statek/1 -> Bus Selector3/1
  MATLAB Function2/1(ui_gamma) -> MATLAB Function1/5(ui_gamma)
  Discrete-Time Integrator1/1 -> MATLAB Function1/2(phiAlpha_int)
  Bus Selector2/2 -> Demux11/1, Demux8/1  "<xyz_dot>"
  Demux1/2 -> MATLAB Function/8(yj)
  Demux1/1 -> MATLAB Function/7(xj)
  Demux4/2 -> MATLAB Function/2(yi), MATLAB Function2/2(yi), MATLAB Function3/2(yi)
  Demux4/1 -> MATLAB Function/1(xi), MATLAB Function2/1(xi), MATLAB Function3/1(xi)
  Bus Selector2/1 -> Demux1/1, Demux9/1  "<xyz>"
  statej/1 -> Bus Selector2/1
  Demux6/2 -> MATLAB Function2/11(vyr)
  Demux6/1 -> MATLAB Function2/10(vxr)
  Bus Selector/1 -> Demux5/1  "<xi_d>"
  Bus Selector/2 -> Demux6/1  "<dxi_d>"
  state/1 -> Bus Selector1/1
  ref/1 -> Bus Selector/1

== matlab function test_flock_gazebo/MATLAB Function ==
  data: data input; y output
function y = fcn(data)

DATA = data(1:20);
d1 = DATA(1);
d2 = DATA(2);
d3 = DATA(3);
y = [d1;d2;d3];

== matlab function test_flock_gazebo/Virtual_leader ==
  data: t input; xi_d output; dxi_d output; Xd input
function [xi_d, dxi_d]  = fcn(t, Xd)
%#codegen



f=1/110;    %freq in Hz
radius=0.7;   %radius in meters
f2 = 1/35;
radius2 = 1;
sel=2;      %inputs or parameters dont work! only local vars ...

if sel == 1
    if t < 50
       xd     =  0;
       xdotd  =  0;
           
       yd     = 0;
       ydotd  = 0;
           
       zd     = 2;  
       zdotd  = 0; 
           
       xi_d =[xd; yd; zd];
       dxi_d=[xdotd; ydotd; zdotd]; 
       
    elseif t < 80
        xd     =  1;
        xdotd  =  0;
            
        yd     = -1;
        ydotd  = 0;
            
        zd     = 2;  
        zdotd  = 0; 
            
        xi_d =[xd; yd; zd];
        dxi_d=[xdotd; ydotd; zdotd]; 
        
    else
       xd     = radius*sin(2*pi*f*t);
       xdotd  = radius*2*pi*f*cos(2*pi*f*t);
            
       yd     = radius*cos(2*pi*f*t);
       ydotd  = -radius*2*pi*f*sin(2*pi*f*t);
            
       zd     = 3;  %radius*cos(2*pi*f*t) + 5;
       zdotd  = 0;  %-radius*2*pi*f*sin(2*pi*f*t);
           
       xi_d =[xd; yd; zd];
       dxi_d=[xdotd; ydotd; zdotd];
       
    end
end

 if(sel==2)
     xd     =  Xd(1);
     xdotd  =  0;
          
     yd     = Xd(2);
     ydotd  = 0;
          
     zd     = Xd(3);  
     zdotd  = 0; 
          
     xi_d =[xd; yd; zd];
     dxi_d=[xdotd; ydotd; zdotd]; 
     
 end

== matlab function test_flock_gazebo/Translational Control2/Flocking1/MATLAB Function ==
  data: xi input; yi input; zi input; vxi input; vyi input; vzi input; phiAlpha output; aie output; aive output; xj input; yj input; zj input; vxj input; vyj input; vzj input; xk input; yk input; zk input; vxk input; vyk input; vzk input; xl input; yl input; zl input; vxl input; vyl input; vzl input; epsilon parameter; a parameter; b parameter; c parameter; d parameter; e parameter; h parameter

function [phiAlpha, aie, aive]  = phiAlphaFcn(xi, yi, zi, vxi, vyi, vzi, xj, yj, zj, vxj, vyj, vzj, xk, yk, zk, vxk, vyk, vzk, xl, yl, zl, vxl, vyl, vzl, epsilon, a, b, c, d, e, h)
    
    % Flocking parameters
    cAlpha = sigmaNormFun(c, epsilon) ;
    dAlpha = sigmaNormFun(d, epsilon) ;

    %%
    Pi = [xi;yi;zi] ;
    Pj = [xj;yj;zj] ;
    Pk = [xk;yk;zk] ;
    Pl = [xl;yl;zl] ;

    Vi = [vxi;vyi;vzi] ;
    Vj = [vxj;vyj;vzj] ;
    Vk = [vxk;vyk;vzk] ;
    Vl = [vxl;vyl;vzl] ;
            
    %%
    sigmaNormj = sigmaNormFun(Pj - Pi, epsilon) ;
    nij = gradSigmaFun(Pj - Pi, epsilon) ;
    
    sigmaNormk = sigmaNormFun(Pk - Pi, epsilon) ;
    nik = gradSigmaFun(Pk - Pi, epsilon) ;

    sigmaNorml = sigmaNormFun(Pl - Pi, epsilon) ;
    nil = gradSigmaFun(Pl - Pi, epsilon) ;

    %%
    sigma1j = sigma1Fun(sigmaNormj - dAlpha + e) ;
    sigma1k = sigma1Fun(sigmaNormk - dAlpha + e) ;
    sigma1l = sigma1Fun(sigmaNorml - dAlpha + e) ;
            
    %% Position
    phiAlphaj = 0.5 * bumpFcn(sigmaNormj/cAlpha,h) * ((a+b)*sigma1j + (a-b)) ;
    phiAlphanij = phiAlphaj.* nij ;
    
    phiAlphak = 0.5 * bumpFcn(sigmaNormk/cAlpha,h) * ((a+b)*sigma1k + (a-b)) ;
    phiAlphanik = phiAlphak.* nik ;

    phiAlphal = 0.5 * bumpFcn(sigmaNorml/cAlpha,h) * ((a+b)*sigma1l + (a-b)) ;
    phiAlphanil = phiAlphal.* nil ;

    phiAlpha = phiAlphanij + phiAlphanik + phiAlphanil;

    %
    aije = bumpFcn(sigmaNormj/cAlpha,h).*(Pj - Pi);

    aike = bumpFcn(sigmaNormj/cAlpha,h).*(Pk - Pi);

    aile = bumpFcn(sigmaNorml/cAlpha,h).*(Pl - Pi);

    aie = aije + aike + aile;

    %% Velocity
    aijve = bumpFcn(sigmaNormj/cAlpha,h).*(Vj - Vi);

    aikve = bumpFcn(sigmaNormk/cAlpha,h).*(Vk - Vi);

    ailve = bumpFcn(sigmaNorml/cAlpha,h).*(Vl - Vi);

    aive = aijve + aikve + ailve;
    
end

== matlab function test_flock_gazebo/Translational Control2/Flocking1/MATLAB Function1 ==
  data: phiAlpha input; phiAlpha_int input; aie input; aive input; ui_gamma input; yaw input; Ui_pos output size=3; KP parameter; ui_yaw output

function [Ui_pos, ui_yaw]  = ctrlLaw(phiAlpha, phiAlpha_int, aie, aive, ui_gamma, yaw, KP)  %, phiBetak, bikobs, phiBetanei, bikve
    
    head = yaw(1:2);
    headp = head(1);
    headd = head(2);

    % Control gains and parameters
    Kx = KP(1); Ky = KP(2); Kz = KP(3);
    Kpx = KP(4); Kpy = KP(5); Kpz = KP(6);
    Kdx = KP(7); Kdy = KP(8); Kdz = KP(9);
    Kix = KP(10); Kiy = KP(11); Kiz = KP(12);
    cBetax = KP(13); cBetay = KP(14); cBetaz = KP(15);
    cdBetax = KP(16); cdBetay = KP(17); cdBetaz = KP(18);
    Kyaw = KP(19); Kdyaw = KP(20);
    
    hx_dot = Kx * phiAlpha(1,1) + Kpx * aie(1,1) + Kdx * aive(1,1) + Kix * phiAlpha_int(1,1) + ui_gamma(1,1);  %+ cBetax * (phiBetak(1,1) + phiBetanei(1,1)) + cdBetax * (bikobs(1,1) + bikve(1,1));
    hy_dot = Ky * phiAlpha(2,1) + Kpy * aie(2,1) + Kdy * aive(2,1) + Kiy * phiAlpha_int(2,1) + ui_gamma(2,1);  %+ cBetay * (phiBetak(2,1) + phiBetanei(2,1)) + cdBetay * (bikobs(2,1) + bikve(2,1));
    hz_dot = Kz * phiAlpha(3,1) + Kpz * aie(3,1) + Kdz * aive(3,1) + Kiz * phiAlpha_int(3,1) + ui_gamma(3,1);  %+ cBetaz * (phiBetak(3,1) + phiBetanei(3,1)) + cdBetaz * (bikobs(3,1) + bikve(3,1));
    

    eyaw = 0 - headp;   evyaw = 0 - headd;
    

    Ui_pos = [hx_dot; hy_dot; hz_dot] ;
    ui_yaw = Kyaw*eyaw + Kdyaw*evyaw;

end

== matlab function test_flock_gazebo/Translational Control2/Flocking1/MATLAB Function2 ==
  data: xi input; yi input; zi input; vxi input; vyi input; vzi input; ui_gamma output; xr input; yr input; zr input; vxr input; vyr input; vzr input; c_gammap parameter; xmin parameter; xmax parameter; c_gammav parameter

function ui_gamma   = naviFeedback(xi, yi, zi, vxi, vyi, vzi, xr, yr, zr, vxr, vyr, vzr, c_gammap, xmin, xmax, c_gammav)
    
       
    Pi = [xi ; yi ; zi] ;
    Vi = [vxi ; vyi ; vzi] ;


    Pr = [xr ; yr ; zr] ;
    Vr = [vxr ; vyr ; vzr] ;
    
    ui_gamma = (-1).* satFcn(c_gammap.*(Pi - Pr), xmin, xmax) + (-1).* satFcn(c_gammav.*(Vi - Vr), xmin, xmax) ;
    
end

== matlab function test_flock_gazebo/Translational Control2/Flocking1/MATLAB Function3 ==
  data: xi input; yi input; zi input; vxi input; vyi input; vzi input; xobs parameter; yobs parameter; zobs parameter; vxobs parameter; vyobs parameter; vzobs parameter; phiBetanik output; R parameter; epsilon parameter; d_prime parameter; h parameter; bikobs output
function [phiBetanik, bikobs] = phiBetaFcn(xi, yi, zi, vxi, vyi, vzi, xobs, yobs, zobs, vxobs, vyobs, vzobs, R, epsilon, d_prime, h)
    
    dBeta = sigmaNormFun(d_prime, epsilon) ;
    
    Pi = [xi ; yi ; zi] ;
    Pc = [xobs ; yobs ; zobs] ;
    
    Vi = [vxi ; vyi ; vzi] ;
    Vc = [vxobs ; vyobs ; vzobs] ;

    % Compute closest point between the robot center and the obstacle
    % circumference (ossumming obstacles are circles)
    Pk = Pc + (Pi - Pc) * (R /norm(Pi - Pc)) ;
    %Pk = [xobs ; yobs] ;
    
    sigmaNormk = sigmaNormFun(Pk - Pi, epsilon) ;
    nik = gradSigmaFun(Pk - Pi, epsilon) ;
    
    sigma1k = sigma1Fun(sigmaNormk - dBeta) ;
    
    %% Position
    phiBetak = bumpFcn(sigmaNormk/dBeta,h) * (sigma1k - 1) ;
    phiBetanik = phiBetak.* nik ;
    
    %% Velocity
    bikobs = bumpFcn(sigmaNormk/dBeta,h).*(Vc + (Vi - Vc));
end

== matlab function test_flock_gazebo/Translational Control2/Flocking1/MATLAB Function4 ==
  data: xj input; yj input; zj input; vxj input; vyj input; vzj input; xk input; yk input; zk input; vxk input; vyk input; vzk input; xl input; yl input; zl input; vxl input; vyl input; vzl input; xobs parameter; yobs parameter; zobs parameter; phiBetaniknei output; R parameter; epsilon parameter; d_prime parameter; h parameter; vxobs parameter; vyobs parameter; vzobs parameter; bikve output
function [phiBetaniknei, bikve] = phiBetaFcn(xj, yj, zj, vxj, vyj, vzj, xk, yk, zk, vxk, vyk, vzk, xl, yl, zl, vxl, vyl, vzl, xobs, yobs, zobs, R, epsilon, d_prime, h, vxobs, vyobs, vzobs)
    
    dBeta = sigmaNormFun(d_prime, epsilon) ;
    
    Pj = [xj ; yj ; zj] ;
    Pk = [xk ; yk ; zk] ;
    Pl = [xl ; yl ; zl] ;
    Pc = [xobs ; yobs ; zobs] ;

    Vj = [vxj ; vyj ; vzj] ;
    Vk = [vxk ; vyk ; vzk] ;
    Vl = [vxl ; vyl ; vzl] ;
    Vc = [vxobs ; vyobs ; vzobs] ;

    % Compute closest point between the robot center and the obstacle
    % circumference (ossumming obstacles are circles)
    Pobsj = Pc + (Pj - Pc) * (R /norm(Pj - Pc)) ;
    Pobsk = Pc + (Pk - Pc) * (R /norm(Pk - Pc)) ;
    Pobsl = Pc + (Pl - Pc) * (R /norm(Pl - Pc)) ;
    %Pk = [xobs ; yobs] ;
    
    %%
    sigmaNormj = sigmaNormFun(Pobsj - Pj, epsilon) ;
    nij = gradSigmaFun(Pobsj - Pj, epsilon) ;
    
    sigmaNormk = sigmaNormFun(Pobsk - Pk, epsilon) ;
    nik = gradSigmaFun(Pobsk - Pk, epsilon) ;

    sigmaNorml = sigmaNormFun(Pobsl - Pl, epsilon) ;
    nil = gradSigmaFun(Pobsl - Pl, epsilon) ;

    %%
    sigma1j = sigma1Fun(sigmaNormj - dBeta) ;
    sigma1k = sigma1Fun(sigmaNormk - dBeta) ;
    sigma1l = sigma1Fun(sigmaNorml - dBeta) ;
            
    %%
    phiBetaj = bumpFcn(sigmaNormj/dBeta,h) * (sigma1j - 1) ;
    phiBetak = bumpFcn(sigmaNormk/dBeta,h) * (sigma1k - 1) ;
    phiBetal = bumpFcn(sigmaNorml/dBeta,h) * (sigma1l - 1) ;
            
    %% Position
    phiBetaniknei = phiBetaj.* nij + phiBetak.* nik + phiBetal.* nil;
    
    %% Velocity
    bikve = bumpFcn(sigmaNormj/dBeta,h).*(Vc + (Vj - Vc)) + bumpFcn(sigmaNormk/dBeta,h).*(Vc + (Vk - Vc)) + bumpFcn(sigmaNorml/dBeta,h).*(Vc + (Vl - Vc));
end

== matlab function test_flock_gazebo/Translational Control3/Flocking1/MATLAB Function ==
  data: xi input; yi input; zi input; vxi input; vyi input; vzi input; phiAlpha output; aie output; aive output; xj input; yj input; zj input; vxj input; vyj input; vzj input; xk input; yk input; zk input; vxk input; vyk input; vzk input; xl input; yl input; zl input; vxl input; vyl input; vzl input; epsilon parameter; a parameter; b parameter; c parameter; d parameter; e parameter; h parameter

function [phiAlpha, aie, aive]  = phiAlphaFcn(xi, yi, zi, vxi, vyi, vzi, xj, yj, zj, vxj, vyj, vzj, xk, yk, zk, vxk, vyk, vzk, xl, yl, zl, vxl, vyl, vzl, epsilon, a, b, c, d, e, h)
    
    % Flocking parameters
    cAlpha = sigmaNormFun(c, epsilon) ;
    dAlpha = sigmaNormFun(d, epsilon) ;

    %%
    Pi = [xi;yi;zi] ;
    Pj = [xj;yj;zj] ;
    Pk = [xk;yk;zk] ;
    Pl = [xl;yl;zl] ;

    Vi = [vxi;vyi;vzi] ;
    Vj = [vxj;vyj;vzj] ;
    Vk = [vxk;vyk;vzk] ;
    Vl = [vxl;vyl;vzl] ;
            
    %%
    sigmaNormj = sigmaNormFun(Pj - Pi, epsilon) ;
    nij = gradSigmaFun(Pj - Pi, epsilon) ;
    
    sigmaNormk = sigmaNormFun(Pk - Pi, epsilon) ;
    nik = gradSigmaFun(Pk - Pi, epsilon) ;

    sigmaNorml = sigmaNormFun(Pl - Pi, epsilon) ;
    nil = gradSigmaFun(Pl - Pi, epsilon) ;

    %%
    sigma1j = sigma1Fun(sigmaNormj - dAlpha + e) ;
    sigma1k = sigma1Fun(sigmaNormk - dAlpha + e) ;
    sigma1l = sigma1Fun(sigmaNorml - dAlpha + e) ;
            
    %% Position
    phiAlphaj = 0.5 * bumpFcn(sigmaNormj/cAlpha,h) * ((a+b)*sigma1j + (a-b)) ;
    phiAlphanij = phiAlphaj.* nij ;
    
    phiAlphak = 0.5 * bumpFcn(sigmaNormk/cAlpha,h) * ((a+b)*sigma1k + (a-b)) ;
    phiAlphanik = phiAlphak.* nik ;

    phiAlphal = 0.5 * bumpFcn(sigmaNorml/cAlpha,h) * ((a+b)*sigma1l + (a-b)) ;
    phiAlphanil = phiAlphal.* nil ;

    phiAlpha = phiAlphanij + phiAlphanik + phiAlphanil;

    %
    aije = bumpFcn(sigmaNormj/cAlpha,h).*(Pj - Pi);

    aike = bumpFcn(sigmaNormj/cAlpha,h).*(Pk - Pi);

    aile = bumpFcn(sigmaNorml/cAlpha,h).*(Pl - Pi);

    aie = aije + aike + aile;

    %% Velocity
    aijve = bumpFcn(sigmaNormj/cAlpha,h).*(Vj - Vi);

    aikve = bumpFcn(sigmaNormk/cAlpha,h).*(Vk - Vi);

    ailve = bumpFcn(sigmaNorml/cAlpha,h).*(Vl - Vi);

    aive = aijve + aikve + ailve;
    
end
